simulink model "npc_controller"  (R2022a)
settings: Solver=FixedStepDiscrete  StartTime=0.0  StopTime=20  RelTol=1e-3  EnableMultiTasking=on
undefined symbols (not defined in the file): CAN_O_INT, CANA_BASE, Down, GPTRIP1SEL, GPTRIP2SEL, GPTRIP3SEL, Tsw, TZ1, TZ2, TZ3, Up
libraries: simulink x147, hdlsllib x90, c2802xlib x34, c2837xDlib x20, c280xlib x12, canmsglib x9, c2838xlib x8, idelinklib_common x3, c2806xlib x2, slpidlib x2, c28004xlib x2, c281xlib x2
(part 36 of 42)

== system npc_controller/CONTROL/STATE-MACHINE/CPU_CONTROL_750_precharge_pfc_ok2/updateSequencePhC/pol_final1/prot/System Outputs ==

== system npc_controller/CONTROL/STATE-MACHINE/CPU_CONTROL_750_precharge_pfc_ok2/updateSequencePhC/pol_vxn1/neg/System Outputs1 ==

== system npc_controller/CONTROL/STATE-MACHINE/CPU_CONTROL_750_precharge_pfc_ok2/updateSequencePhC/pol_vxn1/pos/System Outputs1 ==

== system npc_controller/CONTROL/STATE-MACHINE/CPU_CONTROL_750_precharge_pfc_ok2/updateSequencePhC/pol_vxn1/zero/System Outputs1 ==

== system npc_controller/CONTROL/SVPWM/PLL_Block/SRF_PLL/Integrator/Accumulation ==
  In1 : Inport  OutDataTypeStr=single
  Action Port : ActionPort
  Out : Outport  OutDataTypeStr=single
  wires:
  In1/1 -> Out/1

== system npc_controller/CONTROL/SVPWM/PLL_Block/SRF_PLL/Integrator/Reset Integrator ==
  Action Port : ActionPort
  Constant1 : Constant  Value=0  OutDataTypeStr=single
  Out : Outport
  wires:
  Constant1/1 -> Out/1

== system npc_controller/IDLE_AND_TIMER/codegen/CAN_Task/Rx_Handler/ ProcessMB10/All Legs ==
  Action Port : ActionPort  ActionPortLabel=elseif( u1 == 4)
  Data Store Write1 : DataStoreWrite  DataStoreName=u8SinglePhaseLeg  IndexOptions=Index vector (dialog)  Indices=1  OutputSizes=1
  Leg All : Constant  Value=4  OutDataTypeStr=uint8
  wires:
  Leg All/1 -> Data Store Write1/1

== system npc_controller/IDLE_AND_TIMER/codegen/CAN_Task/Rx_Handler/ ProcessMB10/Leg A ==
  Action Port : ActionPort  ActionPortLabel=if(u1 == 1)
  Data Store Write1 : DataStoreWrite  DataStoreName=u8SinglePhaseLeg  IndexOptions=Index vector (dialog)  Indices=1  OutputSizes=1
  Leg A : Constant  OutDataTypeStr=uint8
  wires:
  Leg A/1 -> Data Store Write1/1

== system npc_controller/IDLE_AND_TIMER/codegen/CAN_Task/Rx_Handler/ ProcessMB10/Leg B ==
  Action Port : ActionPort  ActionPortLabel=elseif(u1 == 2)
  Data Store Write1 : DataStoreWrite  DataStoreName=u8SinglePhaseLeg  IndexOptions=Index vector (dialog)  Indices=1  OutputSizes=1
  Leg B : Constant  Value=2  OutDataTypeStr=uint8
  wires:
  Leg B/1 -> Data Store Write1/1

== system npc_controller/IDLE_AND_TIMER/codegen/CAN_Task/Rx_Handler/ ProcessMB10/Leg C ==
  Action Port : ActionPort  ActionPortLabel=elseif( u1 == 3)
  Data Store Write1 : DataStoreWrite  DataStoreName=u8SinglePhaseLeg  IndexOptions=Index vector (dialog)  Indices=1  OutputSizes=1
  Leg C : Constant  Value=3  OutDataTypeStr=uint8
  wires:
  Leg C/1 -> Data Store Write1/1

== system npc_controller/IDLE_AND_TIMER/codegen/CAN_Task/Rx_Handler/ ProcessMB10/Mode_Cmd ==
  Input : Inport
  Action Port : ActionPort  ActionPortLabel=if(u1 == 1)
  Data Store Write1 : DataStoreWrite  DataStoreName=u8ModeCmd  IndexOptions=Index vector (dialog)  Indices=1  OutputSizes=1
  wires:
  Input/1 -> Data Store Write1/1

== system npc_controller/IDLE_AND_TIMER/codegen/CAN_Task/Rx_Handler/ ProcessMB10/Phase Type 1 Phase ==
  Action Port : ActionPort  ActionPortLabel=if(u1 == 1)
  Data Store Write1 : DataStoreWrite  DataStoreName=u8GridPhaseType  IndexOptions=Index vector (dialog)  Indices=1  OutputSizes=1
  Single Phase : Constant  OutDataTypeStr=uint8
  wires:
  Single Phase/1 -> Data Store Write1/1

== system npc_controller/IDLE_AND_TIMER/codegen/CAN_Task/Rx_Handler/ ProcessMB10/Phase Type 3 Phase ==
  Action Port : ActionPort  ActionPortLabel=else
  Data Store Write1 : DataStoreWrite  DataStoreName=u8GridPhaseType  IndexOptions=Index vector (dialog)  Indices=1  OutputSizes=1
  Three Phase : Constant  Value=0  OutDataTypeStr=uint8
  wires:
  Three Phase/1 -> Data Store Write1/1

== system npc_controller/IDLE_AND_TIMER/codegen/CAN_Task/Rx_Handler/ProcessMB11/Red_Mode_Cmd ==
  Input : Inport
  Action Port : ActionPort  ActionPortLabel=if(u1 == 1)
  Data Store Write1 : DataStoreWrite  DataStoreName=u8RedunModeCmd  IndexOptions=Index vector (dialog)  Indices=1  OutputSizes=1
  wires:
  Input/1 -> Data Store Write1/1

== system npc_controller/IDLE_AND_TIMER/codegen/CAN_Task/Rx_Handler/ProcessMB12/Debug_Cmd ==
  Action Port : ActionPort  ActionPortLabel=elseif( u1==2)
  Constant3 : Constant  Value=[1:1]
  Data Store Read1 : DataStoreRead  DataStoreName=u8CanDataRx12  IndexOptions=Index vector (dialog)  Indices=1  OutputSizes=1
  Debug En/Dis : Subsystem  TreatAsAtomicUnit=on
  FUT En Dis : Subsystem  TreatAsAtomicUnit=on
  If1 : If  IfExpression=u1 == hex2dec('0xDA')  ElseIfExpressions=u1 == hex2dec('0xDB')
  Selector3 : Selector  IndexMode=Zero-based  InputPortWidth=8  IndexOptions=Index vector (port)  Indices=[1 3]  OutputSizes=1
  wires:
  If1/2 -> FUT En Dis/Action
  If1/1 -> Debug En/Dis/Action
  Constant3/1 -> Selector3/2
  Data Store Read1/1 -> Selector3/1
  Selector3/1 -> If1/1

== system npc_controller/IDLE_AND_TIMER/codegen/CAN_Task/Rx_Handler/ProcessMB12/Debug_Read ==
  Action Port : ActionPort  ActionPortLabel=if(u1 == 0)
  Constant2 : Constant  Value=[1:1]
  Data Store Read : DataStoreRead  DataStoreName=u8CanDataRx12  IndexOptions=Index vector (dialog)  Indices=1  OutputSizes=1
  Debug_Cmd : Subsystem  TreatAsAtomicUnit=on
  Equal{,1..3} (4 alike) : RelationalOperator  Operator===  OutDataTypeStr=boolean  RndMeth=Simplest  InputSameDT=off
  If : If  IfExpression=u1 == 1
  OR : Logic  Operator=OR  Inputs=4  IconShape=distinctive  AllPortsSameDT=off  OutDataTypeStr=boolean
  RdReq_Calib : Constant  Value=0xD0
  RdReq_Deb1 : Constant  Value=0xD1
  RdReq_Deb2 : Constant  Value=0xD2
  RdReq_FwRev : Constant  Value=0xF0
  Selector1 : Selector  IndexMode=Zero-based  InputPortWidth=8  IndexOptions=Index vector (port)  Indices=[1 3]  OutputSizes=1
  wires:
  Constant2/1 -> Selector1/2
  Data Store Read/1 -> Selector1/1
  RdReq_FwRev/1 -> Equal/2
  RdReq_Calib/1 -> Equal1/2
  Selector1/1 -> Equal1/1, Equal2/1, Debug_Cmd/1(Input), Equal3/1, Equal/1
  RdReq_Deb2/1 -> Equal3/2
  RdReq_Deb1/1 -> Equal2/2
  Equal2/1 -> OR/3
  Equal3/1 -> OR/4
  Equal1/1 -> OR/2
  Equal/1 -> OR/1
  OR/1 -> If/1
  If/1 -> Debug_Cmd/Action

== system npc_controller/IDLE_AND_TIMER/codegen/CAN_Task/Rx_Handler/ProcessMB12/Debug_Write ==
  Action Port : ActionPort  ActionPortLabel=elseif(u1 ==1)

== system npc_controller/IDLE_AND_TIMER/codegen/CAN_Task/Tx_Handler/Run Tx Routine/TxReadRequest ==
  Action Port : ActionPort  ActionPortLabel=if(u1 == 1 & u2 == 1)
  " Tx FW Rev ID134" : Subsystem  TreatAsAtomicUnit=on
  Constant1 : Constant  Value=0  OutDataTypeStr=boolean
  Data Store Read2 : DataStoreRead  DataStoreName=u8RdReqMsgPntr  IndexOptions=Index vector (dialog)  Indices=1  OutputSizes=1
  Data Store Write1 : DataStoreWrite  DataStoreName=b01_ReadRequest  IndexOptions=Index vector (dialog)  Indices=1  OutputSizes=1
  Switch Case : SwitchCase  CaseConditions={0xF0, 0xD0, 0xD1, 0xD2}  ShowDefaultCase=off
  Tx Cal Data ID135 : Subsystem  TreatAsAtomicUnit=on
  Tx TxDeb Dat1 136 : Subsystem  TreatAsAtomicUnit=on
  Tx TxDeb Dat2 137 : Subsystem  TreatAsAtomicUnit=on
  wires:
  Data Store Read2/1 -> Switch Case/1
  Switch Case/1 -> " Tx FW Rev ID134"/Action
  Switch Case/2 -> Tx Cal Data ID135/Action
  Switch Case/3 -> Tx TxDeb Dat1 136/Action
  Switch Case/4 -> Tx TxDeb Dat2 137/Action
  Constant1/1 -> Data Store Write1/1

== system npc_controller/IDLE_AND_TIMER/codegen/CAN_Task/Tx_Handler/Run Tx Routine/TxStatusData ==
  Action Port : ActionPort  ActionPortLabel=else
  Data Store Read2 : DataStoreRead  DataStoreName=u8CanTxIndex  IndexOptions=Index vector (dialog)  Indices=1  OutputSizes=1
  Switch Case : SwitchCase  CaseConditions={0, 1, 2, 3, 4}  ShowDefaultCase=off
  Tx Pri Status ID110 : Subsystem  TreatAsAtomicUnit=on
  Tx Pri1 ID130 : Subsystem  TreatAsAtomicUnit=on
  Tx Pri2 ID131 : Subsystem  TreatAsAtomicUnit=on
  Tx Pri3 ID132 : Subsystem  TreatAsAtomicUnit=on
  Tx Pri4 ID133 : Subsystem  TreatAsAtomicUnit=on
  wires:
  Data Store Read2/1 -> Switch Case/1
  Switch Case/1 -> Tx Pri Status ID110/Action
  Switch Case/2 -> Tx Pri1 ID130/Action
  Switch Case/3 -> Tx Pri2 ID131/Action
  Switch Case/4 -> Tx Pri3 ID132/Action
  Switch Case/5 -> Tx Pri4 ID133/Action

== system npc_controller/IDLE_AND_TIMER/codegen/IDLE/idle_task/get_adc_tmp_mux/get_tmp_mux_inlet ==
  In1 : Inport
  Action Port : ActionPort  ActionPortLabel=case [ 3 ]:
  Data Store Write13 : DataStoreWrite  DataStoreName=adc_temp_inlet  IndexOptions=Index vector (dialog)  Indices=1  OutputSizes=1
  wires:
  In1/1 -> Data Store Write13/1

== system npc_controller/IDLE_AND_TIMER/codegen/IDLE/idle_task/get_adc_tmp_mux/get_tmp_mux_npca ==
  In1 : Inport
  Action Port : ActionPort  ActionPortLabel=case [ 0 ]:
  Data Store Write13 : DataStoreWrite  DataStoreName=adc_temp_npca  IndexOptions=Index vector (dialog)  Indices=1  OutputSizes=1
  wires:
  In1/1 -> Data Store Write13/1

== system npc_controller/IDLE_AND_TIMER/codegen/IDLE/idle_task/get_adc_tmp_mux/get_tmp_mux_npcb ==
  In1 : Inport
  Action Port : ActionPort  ActionPortLabel=case [ 1 ]:
  Data Store Write13 : DataStoreWrite  DataStoreName=adc_temp_npcb  IndexOptions=Index vector (dialog)  Indices=1  OutputSizes=1
  wires:
  In1/1 -> Data Store Write13/1

== system npc_controller/IDLE_AND_TIMER/codegen/IDLE/idle_task/get_adc_tmp_mux/get_tmp_mux_npcc ==
  In1 : Inport
  Action Port : ActionPort  ActionPortLabel=case [ 2 ]:
  Data Store Write13 : DataStoreWrite  DataStoreName=adc_temp_npcc  IndexOptions=Index vector (dialog)  Indices=1  OutputSizes=1
  wires:
  In1/1 -> Data Store Write13/1

== system npc_controller/IDLE_AND_TIMER/codegen/IDLE/idle_task/hkeep/tfv ==
  function : TriggerPort  TriggerType=function-call  VariantControl=Variant
  hkeep1 : Stateflow chart  TreatAsAtomicUnit=on

== system npc_controller/IDLE_AND_TIMER/codegen/IDLE/idle_task/hkeep/tz ==
  note: Reading the trip zone flag from epwm2 and writing to tz_ocp and tz_ovp flags
  note: npc_controller_DWork .tz_ocp = EPwm2Regs.TZOSTFLG.bit.OST1;
      | npc_controller_DWork .tz_ovp = EPwm2Regs.TZOSTFLG.bit.OST2;
      |
      | /*npc_controller_DWork .tz_cmpssocp = EPwm2Regs.TZOSTFLG.bit.DCAEVT1 | EPwm2Regs.TZOSTFLG.bit.DCBEVT1 | EPwm7Regs.TZOSTFLG.bit.DCAEVT1 | EPwm7Regs.TZOSTFLG.bit.DCBEVT1 | EPwm8Regs.TZOSTFLG.bit.DCAEVT1 | EPwm8Regs.TZOSTFLG.bit.DCBEVT1 | EPwm9Regs.TZOSTFLG.bit.DCAEVT1 | EPwm9Regs.TZOSTFLG.bit.DCBEVT1| EPwm10Regs.TZOSTFLG.bit.DCAEVT1 | EPwm10Regs.TZOSTFLG.bit.DCBEVT1 | EPwm11Regs.TZOSTFLG.bit.DCAEVT1 | EPwm11Regs.TZOSTFLG.bit.DCBEVT1;*/
      |
      | /*npc_controller_DWork .tz_cmpssocp = EPwm2Regs.TZFLG.bit.DCAEVT1 | EPwm2Regs.TZFLG.bit.DCBEVT1 | EPwm7Regs.TZFLG.bit.DCAEVT1 | EPwm7Regs.TZFLG.bit.DCBEVT1 | EPwm8Regs.TZFLG.bit.DCAEVT1 | EPwm8Regs.TZFLG.bit.DCBEVT1 | EPwm9Regs.TZFLG.bit.DCAEVT1 | EPwm9Regs.TZFLG.bit.DCBEVT1| EPwm10Regs.TZFLG.bit.DCAEVT1 | EPwm10Regs.TZFLG.bit.DCBEVT1 | EPwm11Regs.TZFLG.bit.DCAEVT1 | EPwm11Regs.TZFLG.bit.DCBEVT1;*/
      |
      | /*npc_controller_DWork .tz_ocp = EPwm7Regs.TZOSTFLG.bit.OST1;
      | npc_controller_DWork .tz_ovp = EPwm7Regs.TZOSTFLG.bit.OST2;
      |
      | npc_controller_DWork .tz_ocp = EPwm8Regs.TZOSTFLG.bit.OST1;
      | npc_controller_DWork .tz_ovp = EPwm8Regs.TZOSTFLG.bit.OST2;
      |
      | npc_controller_DWork .tz_ocp = EPwm9Regs.TZOSTFLG.bit.OST1;
      | npc_controller_DWork .tz_ovp = EPwm9Regs.TZOSTFLG.bit.OST2;
      |
      | npc_controller_DWork .tz_ocp = EPwm10Regs.TZOSTFLG.bit.OST1;
      | npc_controller_DWork .tz_ovp = EPwm10Regs.TZOSTFLG.bit.OST2;
      |
      | npc_controller_DWork .tz_ocp = EPwm11Regs.TZOSTFLG.bit.OST1;
      | npc_controller_DWork .tz_ovp = EPwm11Regs.TZOSTFLG.bit.OST2;*/
  function : TriggerPort  TriggerType=function-call  VariantControl=Variant
  System Outputs2 : Subsystem  mask(System Outputs){ShowInLibBrowser=0}
      mask prompts: ShowInLibBrowser "Simulink:masks:CustCodeMaskParam1_MP"
      settings: CopyFcn=cccopyfcn(gcb)  OpenFcn=ccopenfcn('System Outputs Function')
      mask Help: eval('feval(''rtwprivate'',''rtwhelpview'',''rtw_sys_outputs_block'')');
      mask Display: disp('System\nOutputs');

== system npc_controller/IDLE_AND_TIMER/codegen/IDLE/idle_task/hkeep/tz1 ==
  note: npc_controller_DWork .tz_ocp = EPwm2Regs.TZOSTFLG.bit.OST1;
      | npc_controller_DWork .tz_ovp = EPwm2Regs.TZOSTFLG.bit.OST2;
      |
      | /*npc_controller_DWork .tz_ocp = EPwm7Regs.TZOSTFLG.bit.OST1;
      | npc_controller_DWork .tz_ovp = EPwm7Regs.TZOSTFLG.bit.OST2;
      |
      | npc_controller_DWork .tz_ocp = EPwm8Regs.TZOSTFLG.bit.OST1;
      | npc_controller_DWork .tz_ovp = EPwm8Regs.TZOSTFLG.bit.OST2;
      |
      | npc_controller_DWork .tz_ocp = EPwm9Regs.TZOSTFLG.bit.OST1;
      | npc_controller_DWork .tz_ovp = EPwm9Regs.TZOSTFLG.bit.OST2;
      |
      | npc_controller_DWork .tz_ocp = EPwm10Regs.TZOSTFLG.bit.OST1;
      | npc_controller_DWork .tz_ovp = EPwm10Regs.TZOSTFLG.bit.OST2;
      |
      | npc_controller_DWork .tz_ocp = EPwm11Regs.TZOSTFLG.bit.OST1;
      | npc_controller_DWork .tz_ovp = EPwm11Regs.TZOSTFLG.bit.OST2;*/
  note: Reading the trip zone flag from epwm2 and writing to tz_ocp and tz_ovp flags
  function : TriggerPort  TriggerType=function-call  VariantControl=Variant
  System Outputs2 : Subsystem  mask(System Outputs){ShowInLibBrowser=0}
      mask prompts: ShowInLibBrowser "Simulink:masks:CustCodeMaskParam1_MP"
      settings: CopyFcn=cccopyfcn(gcb)  OpenFcn=ccopenfcn('System Outputs Function')
      mask Help: eval('feval(''rtwprivate'',''rtwhelpview'',''rtw_sys_outputs_block'')');
      mask Display: disp('System\nOutputs');

== system npc_controller/IDLE_AND_TIMER/codegen/IDLE/idle_task/report_adc/Subsystem1 ==
  adc : Inport
  zero_offset : Inport  Port=2
  gain : Inport  Port=3
  Product6 : Product  OutDataTypeStr=single
  Saturation : Saturate  UpperLimit=inf  LowerLimit=0
  Subtract : Sum  Inputs=+-  AccumDataTypeStr=single  OutDataTypeStr=single
  actual : Outport
  wires:
  Saturation/1 -> Product6/1
  Subtract/1 -> Saturation/1
  zero_offset/1 -> Subtract/2
  adc/1 -> Subtract/1
  gain/1 -> Product6/2
  Product6/1 -> actual/1

== system npc_controller/IDLE_AND_TIMER/codegen/IDLE/idle_task/report_adc/Subsystem10 ==
  adc : Inport
  gain : Inport  Port=2
  Product6 : Product  OutDataTypeStr=single
  actual : Outport
  wires:
  Product6/1 -> actual/1
  gain/1 -> Product6/2
  adc/1 -> Product6/1

== system npc_controller/IDLE_AND_TIMER/codegen/IDLE/idle_task/report_adc/Subsystem11 ==
  adc : Inport
  zero_offset : Inport  Port=2
  gain : Inport  Port=3
  Product6 : Product  OutDataTypeStr=single
  Saturation : Saturate  UpperLimit=inf  LowerLimit=0
  Subtract : Sum  Inputs=+-  AccumDataTypeStr=single  OutDataTypeStr=single
  actual : Outport
  wires:
  Product6/1 -> actual/1
  gain/1 -> Product6/2
  adc/1 -> Subtract/1
  zero_offset/1 -> Subtract/2
  Subtract/1 -> Saturation/1
  Saturation/1 -> Product6/1

== system npc_controller/IDLE_AND_TIMER/codegen/IDLE/idle_task/report_adc/Subsystem2 ==
  adc : Inport
  zero_offset : Inport  Port=2
  gain : Inport  Port=3
  Product6 : Product  OutDataTypeStr=single
  Saturation : Saturate  UpperLimit=inf  LowerLimit=0
  Subtract : Sum  Inputs=+-  AccumDataTypeStr=single  OutDataTypeStr=single
  actual : Outport
  wires:
  Product6/1 -> actual/1
  gain/1 -> Product6/2
  adc/1 -> Subtract/1
  zero_offset/1 -> Subtract/2
  Subtract/1 -> Saturation/1
  Saturation/1 -> Product6/1

== system npc_controller/IDLE_AND_TIMER/codegen/IDLE/idle_task/report_adc/Subsystem3 ==
  adc : Inport
  zero_offset : Inport  Port=2
  gain : Inport  Port=3
  Product6 : Product  OutDataTypeStr=single
  Saturation : Saturate  UpperLimit=inf  LowerLimit=0
  Subtract : Sum  Inputs=+-  AccumDataTypeStr=single  OutDataTypeStr=single
  actual : Outport
  wires:
  Saturation/1 -> Product6/1
  Subtract/1 -> Saturation/1
  zero_offset/1 -> Subtract/2
  adc/1 -> Subtract/1
  gain/1 -> Product6/2
  Product6/1 -> actual/1

== system npc_controller/IDLE_AND_TIMER/codegen/IDLE/idle_task/report_adc/Subsystem4 ==
  adc : Inport
  zero_offset : Inport  Port=2
  gain : Inport  Port=3
  Product6 : Product  OutDataTypeStr=single
  Saturation : Saturate  UpperLimit=inf  LowerLimit=0
  Subtract : Sum  Inputs=+-  AccumDataTypeStr=single  OutDataTypeStr=single
  actual : Outport
  wires:
  Product6/1 -> actual/1
  gain/1 -> Product6/2
  adc/1 -> Subtract/1
  zero_offset/1 -> Subtract/2
  Subtract/1 -> Saturation/1
  Saturation/1 -> Product6/1

== system npc_controller/IDLE_AND_TIMER/codegen/IDLE/idle_task/report_adc/Subsystem5 ==
  adc : Inport
  zero_offset : Inport  Port=2
  gain : Inport  Port=3
  Product6 : Product  OutDataTypeStr=single
  Saturation : Saturate  UpperLimit=inf  LowerLimit=0
  Subtract : Sum  Inputs=+-  AccumDataTypeStr=single  OutDataTypeStr=single
  actual : Outport
  wires:
  Saturation/1 -> Product6/1
  Subtract/1 -> Saturation/1
  zero_offset/1 -> Subtract/2
  adc/1 -> Subtract/1
  gain/1 -> Product6/2
  Product6/1 -> actual/1

== system npc_controller/IDLE_AND_TIMER/codegen/IDLE/idle_task/report_adc/Subsystem6 ==
  adc : Inport
  zero_offset : Inport  Port=2
  gain : Inport  Port=3
  Product6 : Product  OutDataTypeStr=single
  Saturation : Saturate  UpperLimit=inf  LowerLimit=0
  Subtract : Sum  Inputs=+-  AccumDataTypeStr=single  OutDataTypeStr=single
  actual : Outport
  wires:
  Product6/1 -> actual/1
  gain/1 -> Product6/2
  adc/1 -> Subtract/1
  zero_offset/1 -> Subtract/2
  Subtract/1 -> Saturation/1
  Saturation/1 -> Product6/1

== system npc_controller/IDLE_AND_TIMER/codegen/IDLE/idle_task/report_adc/Subsystem7 ==
  adc : Inport
  zero_offset : Inport  Port=2
  gain : Inport  Port=3
  Product6 : Product  OutDataTypeStr=single
  Saturation : Saturate  UpperLimit=inf  LowerLimit=0
  Subtract : Sum  Inputs=+-  AccumDataTypeStr=single  OutDataTypeStr=single
  actual : Outport
  wires:
  Product6/1 -> actual/1
  gain/1 -> Product6/2
  adc/1 -> Subtract/1
  zero_offset/1 -> Subtract/2
  Subtract/1 -> Saturation/1
  Saturation/1 -> Product6/1

== system npc_controller/IDLE_AND_TIMER/codegen/IDLE/idle_task/report_adc/Subsystem8 ==
  adc : Inport
  zero_offset : Inport  Port=2
  gain : Inport  Port=3
  Product6 : Product  OutDataTypeStr=single
  Saturation : Saturate  UpperLimit=inf  LowerLimit=0
  Subtract : Sum  Inputs=+-  AccumDataTypeStr=single  OutDataTypeStr=single
  actual : Outport
  wires:
  Saturation/1 -> Product6/1
  Subtract/1 -> Saturation/1
  zero_offset/1 -> Subtract/2
  adc/1 -> Subtract/1
  gain/1 -> Product6/2
  Product6/1 -> actual/1

== system npc_controller/IDLE_AND_TIMER/codegen/IDLE/idle_task/report_adc/Subsystem9 ==
  adc : Inport
  gain : Inport  Port=2
  Product6 : Product  OutDataTypeStr=single
  actual : Outport
  wires:
  adc/1 -> Product6/1
  gain/1 -> Product6/2
  Product6/1 -> actual/1

== system npc_controller/IDLE_AND_TIMER/codegen/IDLE/idle_task/report_adc1/Subsystem1 ==
  adc : Inport
  zero_offset : Inport  Port=2
  gain : Inport  Port=3
  Product6 : Product  OutDataTypeStr=single
  Saturation : Saturate  UpperLimit=inf  LowerLimit=0
  Subtract : Sum  Inputs=+-  AccumDataTypeStr=single  OutDataTypeStr=single
  actual : Outport
  wires:
  Product6/1 -> actual/1
  gain/1 -> Product6/2
  adc/1 -> Subtract/1
  zero_offset/1 -> Subtract/2
  Subtract/1 -> Saturation/1
  Saturation/1 -> Product6/1

== system npc_controller/IDLE_AND_TIMER/codegen/IDLE/idle_task/report_adc1/Subsystem10 ==
  adc : Inport
  gain : Inport  Port=2
  Product6 : Product  OutDataTypeStr=single
  actual : Outport
  wires:
  adc/1 -> Product6/1
  gain/1 -> Product6/2
  Product6/1 -> actual/1

== system npc_controller/IDLE_AND_TIMER/codegen/IDLE/idle_task/report_adc1/Subsystem11 ==
  adc : Inport
  zero_offset : Inport  Port=2
  gain : Inport  Port=3
  Product6 : Product  OutDataTypeStr=single
  Saturation : Saturate  UpperLimit=inf  LowerLimit=0
  Subtract : Sum  Inputs=+-  AccumDataTypeStr=single  OutDataTypeStr=single
  actual : Outport
  wires:
  Saturation/1 -> Product6/1
  Subtract/1 -> Saturation/1
  zero_offset/1 -> Subtract/2
  adc/1 -> Subtract/1
  gain/1 -> Product6/2
  Product6/1 -> actual/1

== system npc_controller/IDLE_AND_TIMER/codegen/IDLE/idle_task/report_adc1/Subsystem2 ==
  adc : Inport
  zero_offset : Inport  Port=2
  gain : Inport  Port=3
  Product6 : Product  OutDataTypeStr=single
  Saturation : Saturate  UpperLimit=inf  LowerLimit=0
  Subtract : Sum  Inputs=+-  AccumDataTypeStr=single  OutDataTypeStr=single
  actual : Outport
  wires:
  Saturation/1 -> Product6/1
  Subtract/1 -> Saturation/1
  zero_offset/1 -> Subtract/2
  adc/1 -> Subtract/1
  gain/1 -> Product6/2
  Product6/1 -> actual/1

== system npc_controller/IDLE_AND_TIMER/codegen/IDLE/idle_task/report_adc1/Subsystem3 ==
  adc : Inport
  zero_offset : Inport  Port=2
  gain : Inport  Port=3
  Product6 : Product  OutDataTypeStr=single
  Saturation : Saturate  UpperLimit=inf  LowerLimit=0
  Subtract : Sum  Inputs=+-  AccumDataTypeStr=single  OutDataTypeStr=single
  actual : Outport
  wires:
  Product6/1 -> actual/1
  gain/1 -> Product6/2
  adc/1 -> Subtract/1
  zero_offset/1 -> Subtract/2
  Subtract/1 -> Saturation/1
  Saturation/1 -> Product6/1

== system npc_controller/IDLE_AND_TIMER/codegen/IDLE/idle_task/report_adc1/Subsystem4 ==
  adc : Inport
  zero_offset : Inport  Port=2
  gain : Inport  Port=3
  Product6 : Product  OutDataTypeStr=single
  Saturation : Saturate  UpperLimit=inf  LowerLimit=0
  Subtract : Sum  Inputs=+-  AccumDataTypeStr=single  OutDataTypeStr=single
  actual : Outport
  wires:
  Saturation/1 -> Product6/1
  Subtract/1 -> Saturation/1
  zero_offset/1 -> Subtract/2
  adc/1 -> Subtract/1
  gain/1 -> Product6/2
  Product6/1 -> actual/1

== system npc_controller/IDLE_AND_TIMER/codegen/IDLE/idle_task/report_adc1/Subsystem5 ==
  adc : Inport
  zero_offset : Inport  Port=2
  gain : Inport  Port=3
  Product6 : Product  OutDataTypeStr=single
  Saturation : Saturate  UpperLimit=inf  LowerLimit=0
  Subtract : Sum  Inputs=+-  AccumDataTypeStr=single  OutDataTypeStr=single
  actual : Outport
  wires:
  Product6/1 -> actual/1
  gain/1 -> Product6/2
  adc/1 -> Subtract/1
  zero_offset/1 -> Subtract/2
  Subtract/1 -> Saturation/1
  Saturation/1 -> Product6/1

== system npc_controller/IDLE_AND_TIMER/codegen/IDLE/idle_task/report_adc1/Subsystem6 ==
  adc : Inport
  zero_offset : Inport  Port=2
  gain : Inport  Port=3
  Product6 : Product  OutDataTypeStr=single
  Saturation : Saturate  UpperLimit=inf  LowerLimit=0
  Subtract : Sum  Inputs=+-  AccumDataTypeStr=single  OutDataTypeStr=single
  actual : Outport
  wires:
  Saturation/1 -> Product6/1
  Subtract/1 -> Saturation/1
  zero_offset/1 -> Subtract/2
  adc/1 -> Subtract/1
  gain/1 -> Product6/2
  Product6/1 -> actual/1

== system npc_controller/IDLE_AND_TIMER/codegen/IDLE/idle_task/report_adc1/Subsystem7 ==
  adc : Inport
  zero_offset : Inport  Port=2
  gain : Inport  Port=3
  Product6 : Product  OutDataTypeStr=single
  Saturation : Saturate  UpperLimit=inf  LowerLimit=0
  Subtract : Sum  Inputs=+-  AccumDataTypeStr=single  OutDataTypeStr=single
  actual : Outport
  wires:
  Saturation/1 -> Product6/1
  Subtract/1 -> Saturation/1
  zero_offset/1 -> Subtract/2
  adc/1 -> Subtract/1
  gain/1 -> Product6/2
  Product6/1 -> actual/1

== system npc_controller/IDLE_AND_TIMER/codegen/IDLE/idle_task/report_adc1/Subsystem8 ==
  adc : Inport
  zero_offset : Inport  Port=2
  gain : Inport  Port=3
  Product6 : Product  OutDataTypeStr=single
  Saturation : Saturate  UpperLimit=inf  LowerLimit=0
  Subtract : Sum  Inputs=+-  AccumDataTypeStr=single  OutDataTypeStr=single
  actual : Outport
  wires:
  Product6/1 -> actual/1
  gain/1 -> Product6/2
  adc/1 -> Subtract/1
  zero_offset/1 -> Subtract/2
  Subtract/1 -> Saturation/1
  Saturation/1 -> Product6/1

== system npc_controller/IDLE_AND_TIMER/codegen/IDLE/idle_task/report_adc1/Subsystem9 ==
  adc : Inport
  gain : Inport  Port=2
  Product6 : Product  OutDataTypeStr=single
  actual : Outport
  wires:
  Product6/1 -> actual/1
  gain/1 -> Product6/2
  adc/1 -> Product6/1

== system npc_controller/IDLE_AND_TIMER/codegen/IDLE/idle_task/set_tmp_mux/incr_cnt_tmp_mux ==
  function : TriggerPort  TriggerType=function-call  VariantControl=Variant
  Data Store Read : DataStoreRead  DataStoreName=cnt_tmp_mux  IndexOptions=Index vector (dialog)  Indices=1  OutputSizes=1
  If : If  IfExpression=u1 < 4
  cnt_idle : Subsystem  TreatAsAtomicUnit=on
  cnt_idle_sat : Subsystem  TreatAsAtomicUnit=on
  wires:
  Data Store Read/1 -> If/1
  If/1 -> cnt_idle/Action
  If/2 -> cnt_idle_sat/Action

== system npc_controller/IDLE_AND_TIMER/codegen/IDLE/idle_task/set_tmp_mux/parse_cnt_tmp_mux ==
  function : TriggerPort  TriggerType=function-call  VariantControl=Variant
  Data Store Read : DataStoreRead  DataStoreName=cnt_tmp_mux  IndexOptions=Index vector (dialog)  Indices=1  OutputSizes=1
  Switch Case : SwitchCase  CaseConditions={0, 1, 2, 3}
  cnt_tmp_mux_0 : Subsystem  TreatAsAtomicUnit=on
  cnt_tmp_mux_1 : Subsystem  TreatAsAtomicUnit=on
  cnt_tmp_mux_2 : Subsystem  TreatAsAtomicUnit=on
  cnt_tmp_mux_3 : Subsystem  TreatAsAtomicUnit=on
  wires:
  Data Store Read/1 -> Switch Case/1
  Switch Case/1 -> cnt_tmp_mux_0/Action
  Switch Case/2 -> cnt_tmp_mux_1/Action
  Switch Case/3 -> cnt_tmp_mux_2/Action
  Switch Case/4 -> cnt_tmp_mux_3/Action

== system npc_controller/IDLE_AND_TIMER/codegen/IDLE/idle_task/set_tmp_mux/set_tmp_mux ==
  Trigger : TriggerPort  TriggerType=function-call  VariantControl=(inherit)  PortDimensions=1
  Data Store Read : DataStoreRead  DataStoreName=tmp_mux_s0  IndexOptions=Index vector (dialog)  Indices=1  OutputSizes=1
  Data Store Read1 : DataStoreRead  DataStoreName=tmp_mux_s1  IndexOptions=Index vector (dialog)  Indices=1  OutputSizes=1
  Data Store Read2 : DataStoreRead  DataStoreName=tmp_mux_s2  IndexOptions=Index vector (dialog)  Indices=1  OutputSizes=1
  GPIO63 : c2837xDlib/Digital Output  GPIO_Number=GPIO56~GPIO63  GPIO_Bit0=off  GPIO_BIT0_Toggle=off  GPIO_Bit1=off  GPIO_BIT1_Toggle=off  GPIO_Bit2=off  GPIO_BIT2_Toggle=off  GPIO_Bit3=off  GPIO_BIT3_Toggle=off  GPIO_Bit4=off  GPIO_BIT4_Toggle=off  GPIO_Bit5=off  GPIO_BIT5_Toggle=off  GPIO_Bit6=off  GPIO_BIT6_Toggle=off  GPIO_Bit7=on  GPIO_BIT7_Toggle=off
      settings: SourceProductBaseCode=TIC2000
  GPIO64 : c2837xDlib/Digital Output  GPIO_Number=GPIO64~GPIO71  GPIO_Bit0=on  GPIO_BIT0_Toggle=off  GPIO_Bit1=off  GPIO_BIT1_Toggle=off  GPIO_Bit2=off  GPIO_BIT2_Toggle=off  GPIO_Bit3=off  GPIO_BIT3_Toggle=off  GPIO_Bit4=off  GPIO_BIT4_Toggle=off  GPIO_Bit5=off  GPIO_BIT5_Toggle=off  GPIO_Bit6=off  GPIO_BIT6_Toggle=off  GPIO_Bit7=off  GPIO_BIT7_Toggle=off
      settings: SourceProductBaseCode=TIC2000
  GPIO65 : c2837xDlib/Digital Output  GPIO_Number=GPIO64~GPIO71  GPIO_Bit0=off  GPIO_BIT0_Toggle=off  GPIO_Bit1=on  GPIO_BIT1_Toggle=off  GPIO_Bit2=off  GPIO_BIT2_Toggle=off  GPIO_Bit3=off  GPIO_BIT3_Toggle=off  GPIO_Bit4=off  GPIO_BIT4_Toggle=off  GPIO_Bit5=off  GPIO_BIT5_Toggle=off  GPIO_Bit6=off  GPIO_BIT6_Toggle=off  GPIO_Bit7=off  GPIO_BIT7_Toggle=off
      settings: SourceProductBaseCode=TIC2000
  wires:
  Data Store Read1/1 -> GPIO64/1
  Data Store Read/1 -> GPIO63/1
  Data Store Read2/1 -> GPIO65/1

== system npc_controller/IDLE_AND_TIMER/codegen/IDLE/idle_task1/get_adc_tmp_mux/get_tmp_mux_inlet ==
  In1 : Inport
  Action Port : ActionPort  ActionPortLabel=case [ 3 ]:
  Data Store Write13 : DataStoreWrite  DataStoreName=adc_temp_inlet  IndexOptions=Index vector (dialog)  Indices=1  OutputSizes=1
  wires:
  In1/1 -> Data Store Write13/1

== system npc_controller/IDLE_AND_TIMER/codegen/IDLE/idle_task1/get_adc_tmp_mux/get_tmp_mux_npca ==
  In1 : Inport
  Action Port : ActionPort  ActionPortLabel=case [ 0 ]:
  Data Store Write13 : DataStoreWrite  DataStoreName=adc_temp_npca  IndexOptions=Index vector (dialog)  Indices=1  OutputSizes=1
  wires:
  In1/1 -> Data Store Write13/1

== system npc_controller/IDLE_AND_TIMER/codegen/IDLE/idle_task1/get_adc_tmp_mux/get_tmp_mux_npcb ==
  In1 : Inport
  Action Port : ActionPort  ActionPortLabel=case [ 1 ]:
  Data Store Write13 : DataStoreWrite  DataStoreName=adc_temp_npcb  IndexOptions=Index vector (dialog)  Indices=1  OutputSizes=1
  wires:
  In1/1 -> Data Store Write13/1

== system npc_controller/IDLE_AND_TIMER/codegen/IDLE/idle_task1/get_adc_tmp_mux/get_tmp_mux_npcc ==
  In1 : Inport
  Action Port : ActionPort  ActionPortLabel=case [ 2 ]:
  Data Store Write13 : DataStoreWrite  DataStoreName=adc_temp_npcc  IndexOptions=Index vector (dialog)  Indices=1  OutputSizes=1
  wires:
  In1/1 -> Data Store Write13/1

== system npc_controller/IDLE_AND_TIMER/codegen/IDLE/idle_task1/hkeep/tfv ==
  function : TriggerPort  TriggerType=function-call  VariantControl=Variant
  hkeep1 : Stateflow chart  TreatAsAtomicUnit=on

== system npc_controller/IDLE_AND_TIMER/codegen/IDLE/idle_task1/hkeep/tz ==
  note: reading the tz flag through epwm2 registers and writing to tz_ocp and tz_ovp variables. tz_ocp & tz_ovp are used in state machine
  note: npc_controller_DWork .tz_ocp = EPwm2Regs.TZOSTFLG.bit.OST1;
      | npc_controller_DWork .tz_ovp = EPwm2Regs.TZOSTFLG.bit.OST2;
  function : TriggerPort  TriggerType=function-call  VariantControl=Variant
  System Outputs2 : Subsystem  mask(System Outputs){ShowInLibBrowser=0}
      mask prompts: ShowInLibBrowser "Simulink:masks:CustCodeMaskParam1_MP"
      settings: CopyFcn=cccopyfcn(gcb)  OpenFcn=ccopenfcn('System Outputs Function')
      mask Help: eval('feval(''rtwprivate'',''rtwhelpview'',''rtw_sys_outputs_block'')');
      mask Display: disp('System\nOutputs');

== system npc_controller/IDLE_AND_TIMER/codegen/IDLE/idle_task1/report_adc/Subsystem1 ==
  adc : Inport
  zero_offset : Inport  Port=2
  gain : Inport  Port=3
  Product6 : Product  OutDataTypeStr=single
  Saturation : Saturate  UpperLimit=inf  LowerLimit=0
  Subtract : Sum  Inputs=+-  AccumDataTypeStr=single  OutDataTypeStr=single
  actual : Outport
  wires:
  Saturation/1 -> Product6/1
  Subtract/1 -> Saturation/1
  zero_offset/1 -> Subtract/2
  adc/1 -> Subtract/1
  gain/1 -> Product6/2
  Product6/1 -> actual/1

== system npc_controller/IDLE_AND_TIMER/codegen/IDLE/idle_task1/report_adc/Subsystem10 ==
  adc : Inport
  gain : Inport  Port=2
  Product6 : Product  OutDataTypeStr=single
  actual : Outport
  wires:
  Product6/1 -> actual/1
  gain/1 -> Product6/2
  adc/1 -> Product6/1

== system npc_controller/IDLE_AND_TIMER/codegen/IDLE/idle_task1/report_adc/Subsystem11 ==
  adc : Inport
  zero_offset : Inport  Port=2
  gain : Inport  Port=3
  Product6 : Product  OutDataTypeStr=single
  Saturation : Saturate  UpperLimit=inf  LowerLimit=0
  Subtract : Sum  Inputs=+-  AccumDataTypeStr=single  OutDataTypeStr=single
  actual : Outport
  wires:
  Product6/1 -> actual/1
  gain/1 -> Product6/2
  adc/1 -> Subtract/1
  zero_offset/1 -> Subtract/2
  Subtract/1 -> Saturation/1
  Saturation/1 -> Product6/1

== system npc_controller/IDLE_AND_TIMER/codegen/IDLE/idle_task1/report_adc/Subsystem2 ==
  adc : Inport
  zero_offset : Inport  Port=2
  gain : Inport  Port=3
  Product6 : Product  OutDataTypeStr=single
  Saturation : Saturate  UpperLimit=inf  LowerLimit=0
  Subtract : Sum  Inputs=+-  AccumDataTypeStr=single  OutDataTypeStr=single
  actual : Outport
  wires:
  Product6/1 -> actual/1
  gain/1 -> Product6/2
  adc/1 -> Subtract/1
  zero_offset/1 -> Subtract/2
  Subtract/1 -> Saturation/1
  Saturation/1 -> Product6/1

== system npc_controller/IDLE_AND_TIMER/codegen/IDLE/idle_task1/report_adc/Subsystem3 ==
  adc : Inport
  zero_offset : Inport  Port=2
  gain : Inport  Port=3
  Product6 : Product  OutDataTypeStr=single
  Saturation : Saturate  UpperLimit=inf  LowerLimit=0
  Subtract : Sum  Inputs=+-  AccumDataTypeStr=single  OutDataTypeStr=single
  actual : Outport
  wires:
  Saturation/1 -> Product6/1
  Subtract/1 -> Saturation/1
  zero_offset/1 -> Subtract/2
  adc/1 -> Subtract/1
  gain/1 -> Product6/2
  Product6/1 -> actual/1

== system npc_controller/IDLE_AND_TIMER/codegen/IDLE/idle_task1/report_adc/Subsystem4 ==
  adc : Inport
  zero_offset : Inport  Port=2
  gain : Inport  Port=3
  Product6 : Product  OutDataTypeStr=single
  Saturation : Saturate  UpperLimit=inf  LowerLimit=0
  Subtract : Sum  Inputs=+-  AccumDataTypeStr=single  OutDataTypeStr=single
  actual : Outport
  wires:
  Product6/1 -> actual/1
  gain/1 -> Product6/2
  adc/1 -> Subtract/1
  zero_offset/1 -> Subtract/2
  Subtract/1 -> Saturation/1
  Saturation/1 -> Product6/1

== system npc_controller/IDLE_AND_TIMER/codegen/IDLE/idle_task1/report_adc/Subsystem5 ==
  adc : Inport
  zero_offset : Inport  Port=2
  gain : Inport  Port=3
  Product6 : Product  OutDataTypeStr=single
  Saturation : Saturate  UpperLimit=inf  LowerLimit=0
  Subtract : Sum  Inputs=+-  AccumDataTypeStr=single  OutDataTypeStr=single
  actual : Outport
  wires:
  Saturation/1 -> Product6/1
  Subtract/1 -> Saturation/1
  zero_offset/1 -> Subtract/2
  adc/1 -> Subtract/1
  gain/1 -> Product6/2
  Product6/1 -> actual/1

== system npc_controller/IDLE_AND_TIMER/codegen/IDLE/idle_task1/report_adc/Subsystem6 ==
  adc : Inport
  zero_offset : Inport  Port=2
  gain : Inport  Port=3
  Product6 : Product  OutDataTypeStr=single
  Saturation : Saturate  UpperLimit=inf  LowerLimit=0
  Subtract : Sum  Inputs=+-  AccumDataTypeStr=single  OutDataTypeStr=single
  actual : Outport
  wires:
  Product6/1 -> actual/1
  gain/1 -> Product6/2
  adc/1 -> Subtract/1
  zero_offset/1 -> Subtract/2
  Subtract/1 -> Saturation/1
  Saturation/1 -> Product6/1

== system npc_controller/IDLE_AND_TIMER/codegen/IDLE/idle_task1/report_adc/Subsystem7 ==
  adc : Inport
  zero_offset : Inport  Port=2
  gain : Inport  Port=3
  Product6 : Product  OutDataTypeStr=single
  Saturation : Saturate  UpperLimit=inf  LowerLimit=0
  Subtract : Sum  Inputs=+-  AccumDataTypeStr=single  OutDataTypeStr=single
  actual : Outport
  wires:
  Product6/1 -> actual/1
  gain/1 -> Product6/2
  adc/1 -> Subtract/1
  zero_offset/1 -> Subtract/2
  Subtract/1 -> Saturation/1
  Saturation/1 -> Product6/1

== system npc_controller/IDLE_AND_TIMER/codegen/IDLE/idle_task1/report_adc/Subsystem8 ==
  adc : Inport
  zero_offset : Inport  Port=2
  gain : Inport  Port=3
  Product6 : Product  OutDataTypeStr=single
  Saturation : Saturate  UpperLimit=inf  LowerLimit=0
  Subtract : Sum  Inputs=+-  AccumDataTypeStr=single  OutDataTypeStr=single
  actual : Outport
  wires:
  Saturation/1 -> Product6/1
  Subtract/1 -> Saturation/1
  zero_offset/1 -> Subtract/2
  adc/1 -> Subtract/1
  gain/1 -> Product6/2
  Product6/1 -> actual/1

== system npc_controller/IDLE_AND_TIMER/codegen/IDLE/idle_task1/report_adc/Subsystem9 ==
  adc : Inport
  gain : Inport  Port=2
  Product6 : Product  OutDataTypeStr=single
  actual : Outport
  wires:
  adc/1 -> Product6/1
  gain/1 -> Product6/2
  Product6/1 -> actual/1

== system npc_controller/IDLE_AND_TIMER/codegen/IDLE/idle_task1/report_adc1/Subsystem1 ==
  adc : Inport
  zero_offset : Inport  Port=2
  gain : Inport  Port=3
  Product6 : Product  OutDataTypeStr=single
  Saturation : Saturate  UpperLimit=inf  LowerLimit=0
  Subtract : Sum  Inputs=+-  AccumDataTypeStr=single  OutDataTypeStr=single
  actual : Outport
  wires:
  Product6/1 -> actual/1
  gain/1 -> Product6/2
  adc/1 -> Subtract/1
  zero_offset/1 -> Subtract/2
  Subtract/1 -> Saturation/1
  Saturation/1 -> Product6/1

== system npc_controller/IDLE_AND_TIMER/codegen/IDLE/idle_task1/report_adc1/Subsystem10 ==
  adc : Inport
  gain : Inport  Port=2
  Product6 : Product  OutDataTypeStr=single
  actual : Outport
  wires:
  adc/1 -> Product6/1
  gain/1 -> Product6/2
  Product6/1 -> actual/1

== system npc_controller/IDLE_AND_TIMER/codegen/IDLE/idle_task1/report_adc1/Subsystem11 ==
  adc : Inport
  zero_offset : Inport  Port=2
  gain : Inport  Port=3
  Product6 : Product  OutDataTypeStr=single
  Saturation : Saturate  UpperLimit=inf  LowerLimit=0
  Subtract : Sum  Inputs=+-  AccumDataTypeStr=single  OutDataTypeStr=single
  actual : Outport
  wires:
  Saturation/1 -> Product6/1
  Subtract/1 -> Saturation/1
  zero_offset/1 -> Subtract/2
  adc/1 -> Subtract/1
  gain/1 -> Product6/2
  Product6/1 -> actual/1

== system npc_controller/IDLE_AND_TIMER/codegen/IDLE/idle_task1/report_adc1/Subsystem2 ==
  adc : Inport
  zero_offset : Inport  Port=2
  gain : Inport  Port=3
  Product6 : Product  OutDataTypeStr=single
  Saturation : Saturate  UpperLimit=inf  LowerLimit=0
  Subtract : Sum  Inputs=+-  AccumDataTypeStr=single  OutDataTypeStr=single
  actual : Outport
  wires:
  Saturation/1 -> Product6/1
  Subtract/1 -> Saturation/1
  zero_offset/1 -> Subtract/2
  adc/1 -> Subtract/1
  gain/1 -> Product6/2
  Product6/1 -> actual/1

== system npc_controller/IDLE_AND_TIMER/codegen/IDLE/idle_task1/report_adc1/Subsystem3 ==
  adc : Inport
  zero_offset : Inport  Port=2
  gain : Inport  Port=3
  Product6 : Product  OutDataTypeStr=single
  Saturation : Saturate  UpperLimit=inf  LowerLimit=0
  Subtract : Sum  Inputs=+-  AccumDataTypeStr=single  OutDataTypeStr=single
  actual : Outport
  wires:
  Product6/1 -> actual/1
  gain/1 -> Product6/2
  adc/1 -> Subtract/1
  zero_offset/1 -> Subtract/2
  Subtract/1 -> Saturation/1
  Saturation/1 -> Product6/1

== system npc_controller/IDLE_AND_TIMER/codegen/IDLE/idle_task1/report_adc1/Subsystem4 ==
  adc : Inport
  zero_offset : Inport  Port=2
  gain : Inport  Port=3
  Product6 : Product  OutDataTypeStr=single
  Saturation : Saturate  UpperLimit=inf  LowerLimit=0
  Subtract : Sum  Inputs=+-  AccumDataTypeStr=single  OutDataTypeStr=single
  actual : Outport
  wires:
  Saturation/1 -> Product6/1
  Subtract/1 -> Saturation/1
  zero_offset/1 -> Subtract/2
  adc/1 -> Subtract/1
  gain/1 -> Product6/2
  Product6/1 -> actual/1

== system npc_controller/IDLE_AND_TIMER/codegen/IDLE/idle_task1/report_adc1/Subsystem5 ==
  adc : Inport
  zero_offset : Inport  Port=2
  gain : Inport  Port=3
  Product6 : Product  OutDataTypeStr=single
  Saturation : Saturate  UpperLimit=inf  LowerLimit=0
  Subtract : Sum  Inputs=+-  AccumDataTypeStr=single  OutDataTypeStr=single
  actual : Outport
  wires:
  Product6/1 -> actual/1
  gain/1 -> Product6/2
  adc/1 -> Subtract/1
  zero_offset/1 -> Subtract/2
  Subtract/1 -> Saturation/1
  Saturation/1 -> Product6/1

== system npc_controller/IDLE_AND_TIMER/codegen/IDLE/idle_task1/report_adc1/Subsystem6 ==
  adc : Inport
  zero_offset : Inport  Port=2
  gain : Inport  Port=3
  Product6 : Product  OutDataTypeStr=single
  Saturation : Saturate  UpperLimit=inf  LowerLimit=0
  Subtract : Sum  Inputs=+-  AccumDataTypeStr=single  OutDataTypeStr=single
  actual : Outport
  wires:
  Saturation/1 -> Product6/1
  Subtract/1 -> Saturation/1
  zero_offset/1 -> Subtract/2
  adc/1 -> Subtract/1
  gain/1 -> Product6/2
  Product6/1 -> actual/1

== system npc_controller/IDLE_AND_TIMER/codegen/IDLE/idle_task1/report_adc1/Subsystem7 ==
  adc : Inport
  zero_offset : Inport  Port=2
  gain : Inport  Port=3
  Product6 : Product  OutDataTypeStr=single
  Saturation : Saturate  UpperLimit=inf  LowerLimit=0
  Subtract : Sum  Inputs=+-  AccumDataTypeStr=single  OutDataTypeStr=single
  actual : Outport
  wires:
  Saturation/1 -> Product6/1
  Subtract/1 -> Saturation/1
  zero_offset/1 -> Subtract/2
  adc/1 -> Subtract/1
  gain/1 -> Product6/2
  Product6/1 -> actual/1

== system npc_controller/IDLE_AND_TIMER/codegen/IDLE/idle_task1/report_adc1/Subsystem8 ==
  adc : Inport
  zero_offset : Inport  Port=2
  gain : Inport  Port=3
  Product6 : Product  OutDataTypeStr=single
  Saturation : Saturate  UpperLimit=inf  LowerLimit=0
  Subtract : Sum  Inputs=+-  AccumDataTypeStr=single  OutDataTypeStr=single
  actual : Outport
  wires:
  Product6/1 -> actual/1
  gain/1 -> Product6/2
  adc/1 -> Subtract/1
  zero_offset/1 -> Subtract/2
  Subtract/1 -> Saturation/1
  Saturation/1 -> Product6/1

== system npc_controller/IDLE_AND_TIMER/codegen/IDLE/idle_task1/report_adc1/Subsystem9 ==
  adc : Inport
  gain : Inport  Port=2
  Product6 : Product  OutDataTypeStr=single
  actual : Outport
  wires:
  Product6/1 -> actual/1
  gain/1 -> Product6/2
  adc/1 -> Product6/1

== system npc_controller/IDLE_AND_TIMER/codegen/IDLE/idle_task1/set_tmp_mux/incr_cnt_tmp_mux ==
  function : TriggerPort  TriggerType=function-call  VariantControl=Variant
  Data Store Read : DataStoreRead  DataStoreName=cnt_tmp_mux  IndexOptions=Index vector (dialog)  Indices=1  OutputSizes=1
  If : If  IfExpression=u1 < 4
  cnt_idle : Subsystem  TreatAsAtomicUnit=on
  cnt_idle_sat : Subsystem  TreatAsAtomicUnit=on
  wires:
  Data Store Read/1 -> If/1
  If/1 -> cnt_idle/Action
  If/2 -> cnt_idle_sat/Action

== system npc_controller/IDLE_AND_TIMER/codegen/IDLE/idle_task1/set_tmp_mux/parse_cnt_tmp_mux ==
  function : TriggerPort  TriggerType=function-call  VariantControl=Variant
  Data Store Read : DataStoreRead  DataStoreName=cnt_tmp_mux  IndexOptions=Index vector (dialog)  Indices=1  OutputSizes=1
  Switch Case : SwitchCase  CaseConditions={0, 1, 2, 3}
  cnt_tmp_mux_0 : Subsystem  TreatAsAtomicUnit=on
  cnt_tmp_mux_1 : Subsystem  TreatAsAtomicUnit=on
  cnt_tmp_mux_2 : Subsystem  TreatAsAtomicUnit=on
  cnt_tmp_mux_3 : Subsystem  TreatAsAtomicUnit=on
  wires:
  Data Store Read/1 -> Switch Case/1
  Switch Case/1 -> cnt_tmp_mux_0/Action
  Switch Case/2 -> cnt_tmp_mux_1/Action
  Switch Case/3 -> cnt_tmp_mux_2/Action
  Switch Case/4 -> cnt_tmp_mux_3/Action

== system npc_controller/IDLE_AND_TIMER/codegen/IDLE/idle_task1/set_tmp_mux/set_tmp_mux ==
  Trigger : TriggerPort  TriggerType=function-call  VariantControl=(inherit)  PortDimensions=1
  Data Store Read : DataStoreRead  DataStoreName=tmp_mux_s0  IndexOptions=Index vector (dialog)  Indices=1  OutputSizes=1
  Data Store Read1 : DataStoreRead  DataStoreName=tmp_mux_s1  IndexOptions=Index vector (dialog)  Indices=1  OutputSizes=1
  Data Store Read2 : DataStoreRead  DataStoreName=tmp_mux_s2  IndexOptions=Index vector (dialog)  Indices=1  OutputSizes=1
  GPIO63 : c2837xDlib/Digital Output  GPIO_Number=GPIO56~GPIO63  GPIO_Bit0=off  GPIO_BIT0_Toggle=off  GPIO_Bit1=off  GPIO_BIT1_Toggle=off  GPIO_Bit2=off  GPIO_BIT2_Toggle=off  GPIO_Bit3=off  GPIO_BIT3_Toggle=off  GPIO_Bit4=off  GPIO_BIT4_Toggle=off  GPIO_Bit5=off  GPIO_BIT5_Toggle=off  GPIO_Bit6=off  GPIO_BIT6_Toggle=off  GPIO_Bit7=on  GPIO_BIT7_Toggle=off
      settings: SourceProductBaseCode=TIC2000
  GPIO64 : c2837xDlib/Digital Output  GPIO_Number=GPIO64~GPIO71  GPIO_Bit0=on  GPIO_BIT0_Toggle=off  GPIO_Bit1=off  GPIO_BIT1_Toggle=off  GPIO_Bit2=off  GPIO_BIT2_Toggle=off  GPIO_Bit3=off  GPIO_BIT3_Toggle=off  GPIO_Bit4=off  GPIO_BIT4_Toggle=off  GPIO_Bit5=off  GPIO_BIT5_Toggle=off  GPIO_Bit6=off  GPIO_BIT6_Toggle=off  GPIO_Bit7=off  GPIO_BIT7_Toggle=off
      settings: SourceProductBaseCode=TIC2000
  GPIO65 : c2837xDlib/Digital Output  GPIO_Number=GPIO64~GPIO71  GPIO_Bit0=off  GPIO_BIT0_Toggle=off  GPIO_Bit1=on  GPIO_BIT1_Toggle=off  GPIO_Bit2=off  GPIO_BIT2_Toggle=off  GPIO_Bit3=off  GPIO_BIT3_Toggle=off  GPIO_Bit4=off  GPIO_BIT4_Toggle=off  GPIO_Bit5=off  GPIO_BIT5_Toggle=off  GPIO_Bit6=off  GPIO_BIT6_Toggle=off  GPIO_Bit7=off  GPIO_BIT7_Toggle=off
      settings: SourceProductBaseCode=TIC2000
  wires:
  Data Store Read1/1 -> GPIO64/1
  Data Store Read/1 -> GPIO63/1
  Data Store Read2/1 -> GPIO65/1

== system npc_controller/CONTROL/CONTROL/false/CLA_CONTROL/CONTROL/pwm_generation1/Subsystem ==
  note: Note:
      | pol_pha
      | 0 - pos
      | 1 - neg
  pol : Inport
  pwm_s1 : Inport  Port=2
  pwm_s4 : Inport  Port=3
  Cast To Single : DataTypeConversion  OutDataTypeStr=uint8  SaturateOnIntegerOverflow=off  RndMeth=Floor
  If : If  IfExpression=u1 == 0
  If Action Subsystem : Subsystem  TreatAsAtomicUnit=on
  If Action Subsystem1 : Subsystem  TreatAsAtomicUnit=on
  Merge : Merge
  epwm1b : Outport
  wires:
  pol/1 -> Cast To Single/1
  If/2 -> If Action Subsystem1/Action
  If/1 -> If Action Subsystem/Action
  If Action Subsystem1/1(Out1) -> Merge/2
  If Action Subsystem/1(Out1) -> Merge/1
  Merge/1 -> epwm1b/1
  pwm_s1/1 -> If Action Subsystem/1(In1)
  pwm_s4/1 -> If Action Subsystem1/1(In1)
  Cast To Single/1 -> If/1

== system npc_controller/CONTROL/CONTROL/false/CLA_CONTROL/CONTROL/pwm_generation1/Subsystem1 ==
  note: Note:
      | pol_pha
      | 0 - pos
      | 1 - neg
  pol : Inport
  pwm_s1 : Inport  Port=2
  pwm_s4 : Inport  Port=3
  Cast To Single : DataTypeConversion  OutDataTypeStr=uint8  SaturateOnIntegerOverflow=off  RndMeth=Floor
  If : If  IfExpression=u1 == 0
  If Action Subsystem : Subsystem  TreatAsAtomicUnit=on
  If Action Subsystem1 : Subsystem  TreatAsAtomicUnit=on
  Merge : Merge
  epwm1b : Outport
  wires:
  Cast To Single/1 -> If/1
  pwm_s4/1 -> If Action Subsystem1/1(In1)
  pwm_s1/1 -> If Action Subsystem/1(In1)
  Merge/1 -> epwm1b/1
  If Action Subsystem/1(Out1) -> Merge/1
  If Action Subsystem1/1(Out1) -> Merge/2
  If/1 -> If Action Subsystem/Action
  If/2 -> If Action Subsystem1/Action
  pol/1 -> Cast To Single/1

== system npc_controller/CONTROL/CONTROL/false/CLA_CONTROL/CONTROL/pwm_generation1/Subsystem2 ==
  note: Note:
      | pol_pha
      | 0 - pos
      | 1 - neg
  pol : Inport
  pwm_s1 : Inport  Port=2
  pwm_s4 : Inport  Port=3
  Cast To Single : DataTypeConversion  OutDataTypeStr=uint8  SaturateOnIntegerOverflow=off  RndMeth=Floor
  If : If  IfExpression=u1 == 0
  If Action Subsystem : Subsystem  TreatAsAtomicUnit=on
  If Action Subsystem1 : Subsystem  TreatAsAtomicUnit=on
  Merge : Merge
  epwm1b : Outport
  wires:
  pol/1 -> Cast To Single/1
  If/2 -> If Action Subsystem1/Action
  If/1 -> If Action Subsystem/Action
  If Action Subsystem1/1(Out1) -> Merge/2
  If Action Subsystem/1(Out1) -> Merge/1
  Merge/1 -> epwm1b/1
  pwm_s1/1 -> If Action Subsystem/1(In1)
  pwm_s4/1 -> If Action Subsystem1/1(In1)
  Cast To Single/1 -> If/1

== system npc_controller/CONTROL/CONTROL/false/CLA_CONTROL/CONTROL/pwm_generation1/min_duty ==
  cmp : Inport
  Duty0Pct : Subsystem  TreatAsAtomicUnit=on
  Duty5Pct : Subsystem  TreatAsAtomicUnit=on
  If : If  IfExpression=u1 > 76
  Merge : Merge
  cmp_out : Outport
  wires:
  cmp/1 -> Duty5Pct/1(In1), If/1
  Duty0Pct/1(Out1) -> Merge/2
  If/2 -> Duty0Pct/Action
  Duty5Pct/1(Out1) -> Merge/1
  Merge/1 -> cmp_out/1
  If/1 -> Duty5Pct/Action

== system npc_controller/CONTROL/CONTROL/false/CLA_CONTROL/CONTROL/pwm_generation1/min_duty1 ==
  cmp : Inport
  Duty0Pct : Subsystem  TreatAsAtomicUnit=on
  Duty5Pct : Subsystem  TreatAsAtomicUnit=on
  If : If  IfExpression=u1 > 76
  Merge : Merge
  cmp_out : Outport
  wires:
  If/1 -> Duty5Pct/Action
  Merge/1 -> cmp_out/1
  Duty5Pct/1(Out1) -> Merge/1
  If/2 -> Duty0Pct/Action
  Duty0Pct/1(Out1) -> Merge/2
  cmp/1 -> If/1, Duty5Pct/1(In1)

== system npc_controller/CONTROL/CONTROL/false/CLA_CONTROL/CONTROL/pwm_generation1/min_duty2 ==
  cmp : Inport
  Duty0Pct : Subsystem  TreatAsAtomicUnit=on
  Duty5Pct : Subsystem  TreatAsAtomicUnit=on
  If : If  IfExpression=u1 > 76
  Merge : Merge
  cmp_out : Outport
  wires:
  cmp/1 -> Duty5Pct/1(In1), If/1
  Duty0Pct/1(Out1) -> Merge/2
  If/2 -> Duty0Pct/Action
  Duty5Pct/1(Out1) -> Merge/1
  Merge/1 -> cmp_out/1
  If/1 -> Duty5Pct/Action

== system npc_controller/CONTROL/GET_ADC/ADC/codegen/ADCA/Subsystem6/If Action Subsystem ==
  Action Port : ActionPort  ActionPortLabel=if((u1 > 2979) | (u1 < 1525))
  Constant : Constant  OutDataTypeStr=boolean  SampleTime=-1
  Data Store Write1 : DataStoreWrite  DataStoreName=tfv_iphasec  IndexOptions=Index vector (dialog)  Indices=1  OutputSizes=1
  wires:
  Constant/1 -> Data Store Write1/1

== system npc_controller/CONTROL/GET_ADC/ADC/codegen/ADCA/Subsystem6/If Action Subsystem1 ==
  note: +-30Apeak
  note: //3221 = 40A , 1283 = -40A
  Input : Inport
  Action Port : ActionPort  ActionPortLabel=else
  If Action Subsystem : Subsystem  TreatAsAtomicUnit=on
  If1 : If  Commented=on  IfExpression=(u1 > 2979) | (u1 < 1525)
  If2 : If  IfExpression=(u1 > 3221) | (u1 < 1283)
  wires:
  If2/1 -> If Action Subsystem/Action
  Input/1 -> If2/1

== system npc_controller/CONTROL/GET_ADC/ADC/codegen/ADCA/Subsystem6/If Action Subsystem2 ==
  note: -+60Apeak
  Input : Inport
  Action Port : ActionPort  ActionPortLabel=if(u1 == 0)
  If : If  IfExpression=(u1 > 3705) | (u1 < 798)
  If Action Subsystem : Subsystem  TreatAsAtomicUnit=on
  wires:
  Input/1 -> If/1
  If/1 -> If Action Subsystem/Action

== system npc_controller/CONTROL/GET_ADC/ADC/codegen/ADCA/Subsystem6/calib ==
  note: y = 1.0377x - 68.775
  adc : Inport
  Add : Sum  AccumDataTypeStr=single  OutDataTypeStr=single
  Constant1 : Constant  Value=1.0377  OutDataTypeStr=single
  Constant2 : Constant  Value=-68.775  OutDataTypeStr=single
  Product : Product  OutDataTypeStr=single
  adc_calib : Outport
  wires:
  adc/1 -> Product/1
  Constant1/1 -> Product/2
  Product/1 -> Add/1
  Constant2/1 -> Add/2
  Add/1 -> adc_calib/1

== system npc_controller/CONTROL/GET_ADC/ADC/codegen/ADCA/Subsystem7/If Action Subsystem ==
  Action Port : ActionPort  ActionPortLabel=if((u1 > 2979) | (u1 < 1525))
  Constant : Constant  OutDataTypeStr=boolean  SampleTime=-1
  Data Store Write1 : DataStoreWrite  DataStoreName=tfv_iphaseb  IndexOptions=Index vector (dialog)  Indices=1  OutputSizes=1
  wires:
  Constant/1 -> Data Store Write1/1

== system npc_controller/CONTROL/GET_ADC/ADC/codegen/ADCA/Subsystem7/If Action Subsystem1 ==
  note: +-30Apeak
  note: //3221 = 40A , 1283 = -40A
  Input : Inport
  Action Port : ActionPort  ActionPortLabel=else
  If Action Subsystem : Subsystem  TreatAsAtomicUnit=on
  If1 : If  Commented=on  IfExpression=(u1 > 2979) | (u1 < 1525)
  If2 : If  IfExpression=(u1 > 3221) | (u1 < 1283)
  wires:
  If2/1 -> If Action Subsystem/Action
  Input/1 -> If2/1
